simulink model "PFD_tb"  (R2025a)
settings: Solver=VariableStepAuto  StartTime=0.0  StopTime=300e-6  RelTol=1e-3
libraries: msbPllFoundation x2, simulink x2
settings Model: Creator=55479  LastModifiedBy=55479

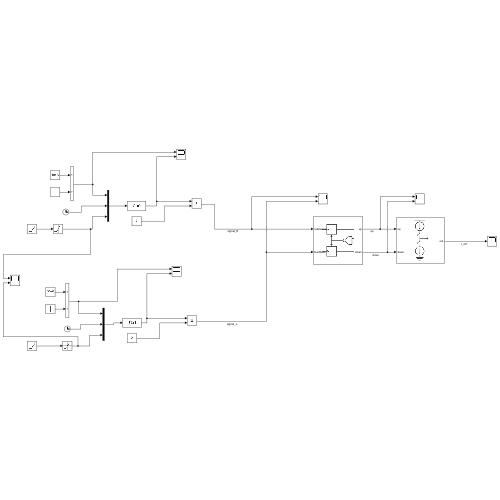
[thumbnail: Simulink's stored preview of the top-level diagram]
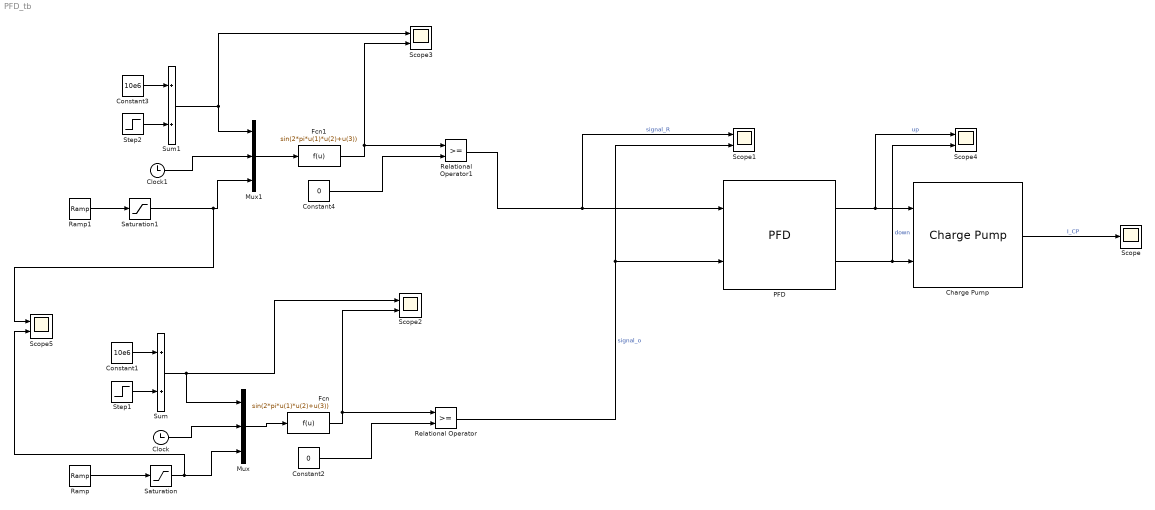
== system PFD_tb ==
  Charge Pump : msbPllFoundation/Charge Pump  OutputCurrent=1e-3  InputThreshold=1e-18  ExtraBuffer=off  NBuffer=1000  EnableCurrentImpairments=off  CurrentImbalance=1e-4  LeakageCurrent=1e-5  EnableTimingImpairments=off  DefaultOrAdvanced=Default  MaxFreqInterest=10e9  RiseFallUp=50e-12  PropDelayUp=60e-12  RiseFallDown=20e-12  PropDelayDown=40e-12
  Clock : Clock
  Clock1 : Clock
  Constant1 : Constant  Value=10e6  SampleTime=1e-9
  Constant2 : Constant  Value=0
  Constant3 : Constant  Value=10e6  SampleTime=1e-9
  Constant4 : Constant  Value=0
  Fcn : Fcn  Expr=sin(2*pi*u(1)*u(2)+u(3))
  Fcn1 : Fcn  Expr=sin(2*pi*u(1)*u(2)+u(3))
  Mux : Mux  Inputs=3
  Mux1 : Mux  Inputs=3
  PFD : msbPllFoundation/PFD  DeadbandCompensation=30e-12  ExtraBuffer=off  NBuffer=1000  EnableImpairments=off  DefaultOrAdvanced=Default  MaxFreqInterest=10e9  RiseFallTime=30e-12  PropDelay=50e-12
  Ramp : simulink/Sources/Ramp  slope=(2 * pi) / 50e-6  start=0  InitialOutput=-3 * (2 * pi)
  Ramp1 : simulink/Sources/Ramp  slope=(2 * pi) / 50e-6  start=3 * 50e-6  InitialOutput=0
  Relational Operator : RelationalOperator  OutDataTypeStr=boolean  RndMeth=Simplest  InputSameDT=off
  Relational Operator1 : RelationalOperator  OutDataTypeStr=boolean  RndMeth=Simplest  InputSameDT=off
  Saturation : Saturate  UpperLimit=0  LowerLimit=-3 * (2 * pi)
  Saturation1 : Saturate  UpperLimit=3 * (2 * pi)  LowerLimit=0
  Scope : Scope
      settings: ActiveDisplayYMinimum=-0.00125  ActiveDisplayYMaximum=0.00125  DataLoggingVariableName=ScopeData2
  Scope{1..5} (5 alike) : Scope  NumInputPorts=2
      Scope1 settings: ActiveDisplayYMinimum=-0.12499999999999997  ActiveDisplayYMaximum=1.125
      Scope2 settings: ActiveDisplayYMinimum=9.875E+6  ActiveDisplayYMaximum=1.1125E+7  DataLoggingVariableName=ScopeData2
      Scope3 settings: ActiveDisplayYMinimum=9.875E+6  ActiveDisplayYMaximum=1.1125E+7  DataLoggingVariableName=ScopeData4
      Scope4 settings: ActiveDisplayYMinimum=-0.12499999999999997  ActiveDisplayYMaximum=1.125  DataLoggingVariableName=ScopeData3
      Scope5 settings: ActiveDisplayYMinimum=-23.561944901923447  ActiveDisplayYMaximum=23.561944901923439  DataLoggingVariableName=ScopeData5
  Step1 : Step  Time=20e-6  After=0  SampleTime=1e-9
  Step2 : Step  Time=20e-6  After=0  SampleTime=1e-9
  Sum : Sum
  Sum1 : Sum
  wires:
  Charge Pump/1 -> Scope/1  "I_CP"
  PFD/2 -> Scope4/2, Charge Pump/2  "down"
  PFD/1 -> Scope4/1, Charge Pump/1  "up"
  Relational Operator/1 -> PFD/2, Scope1/2  "signal_o"
  Step1/1 -> Sum/2
  Constant1/1 -> Sum/1
  Clock/1 -> Mux/2
  Fcn/1 -> Scope2/2, Relational Operator/1
  Constant2/1 -> Relational Operator/2
  Mux/1 -> Fcn/1
  Sum/1 -> Mux/1, Scope2/1
  Relational Operator1/1 -> Scope1/1, PFD/1  "signal_R"
  Saturation/1 -> Scope5/2, Mux/3
  Constant4/1 -> Relational Operator1/2
  Clock1/1 -> Mux1/2
  Constant3/1 -> Sum1/1
  Mux1/1 -> Fcn1/1
  Fcn1/1 -> Scope3/2, Relational Operator1/1
  Step2/1 -> Sum1/2
  Sum1/1 -> Mux1/1, Scope3/1
  Saturation1/1 -> Mux1/3, Scope5/1
  Ramp/1 -> Saturation/1
  Ramp1/1 -> Saturation1/1
